simulink model "SOGI_PLL_NOFLL"  (R2020b)
settings: Solver=FixedStepDiscrete  StartTime=0.0  StopTime=1  FixedStep=1e-6  RelTol=1e-3
undefined symbols (not defined in the file): DiscIntNeverNeededParam
settings Model: Creator=gc45  LastModifiedBy=Administrator

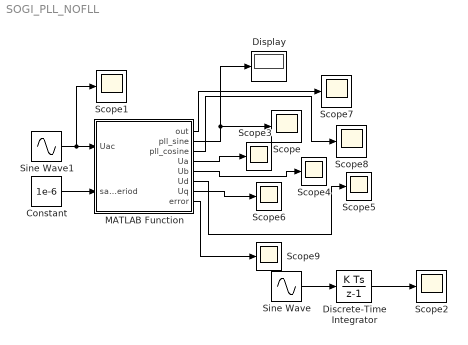
== system SOGI_PLL_NOFLL ==
  Constant : Constant  Value=1e-6
  Discrete-Time Integrator : DiscreteIntegrator  SampleTime=1e-6  ICPrevOutput=DiscIntNeverNeededParam  ICPrevScaledInput=DiscIntNeverNeededParam
  Display : Display
  MATLAB Function : MATLAB Function  TreatAsAtomicUnit=on
  Scope{,1..9} (10 alike) : Scope
  Sine Wave : Sin  Amplitude=100  Frequency=100*pi  SampleTime=1e-6
  Sine Wave1 : Sin  Amplitude=100  Frequency=100*pi  SampleTime=1e-6
  wires:
  Sine Wave1/1 -> Scope1/1, MATLAB Function/1(Uac)
  MATLAB Function/2(pll_sine) -> Display/1, Scope/1
  Constant/1 -> MATLAB Function/2(sample_period)
  Sine Wave/1 -> Discrete-Time Integrator/1
  Discrete-Time Integrator/1 -> Scope2/1
  MATLAB Function/4(Ua) -> Scope3/1
  MATLAB Function/5(Ub) -> Scope4/1
  MATLAB Function/6(Ud) -> Scope5/1
  MATLAB Function/7(Uq) -> Scope6/1
  MATLAB Function/1(out) -> Scope7/1
  MATLAB Function/3(pll_cosine) -> Scope8/1
  MATLAB Function/8(error) -> Scope9/1

== matlab function SOGI_PLL_NOFLL/MATLAB Function ==
  data: out output; Uac input; pll_sine output; sample_period input; pll_cosine output; Ua output; Ub output; Ud output; Uq output; error output
function [out,pll_sine,pll_cosine,Ua,Ub,Ud,Uq,error] = RefGen(Uac, sample_period)

%参数初始化
persistent PredictiveuAC_Intg PredictiveuAC pll_out PhaseDeviation Input_OSG;
persistent pll_Sine pll_Cosine pll_wt Vg_amp PhaseDeviation_Intg;
if isempty(pll_out)
    PredictiveuAC = 0; %Ualpha
	PredictiveuAC_Intg = 0;%Ubeta
	pll_out = 0;
	PhaseDeviation = 0;
	Input_OSG = 0;
	pll_Sine = 0;
	pll_Cosine = 0;
	pll_wt =0;
	Vg_amp = 0;
	PhaseDeviation_Intg = 0;
end
persistent Intg1 Intg2;
if isempty(Intg1)
    Intg1 = 0;
    Intg2 = 0;
end
dataType = 'double';
Kp_Predictive = 1.414;%100>>8
Ki_SOGI = 5;
Kp_SOGI = 15;
%正交信号发生器环节
   Input_OSG = (Uac-PredictiveuAC) * Kp_Predictive;
   Intg1 = (Input_OSG-PredictiveuAC_Intg) * sample_period;
   PredictiveuAC = PredictiveuAC + Intg1 * pll_out;
   Intg2 = PredictiveuAC * sample_period;
   PredictiveuAC_Intg = PredictiveuAC_Intg + Intg2 * pll_out;
%clark变换环节
   PhaseDeviation = PredictiveuAC_Intg*pll_Cosine - PredictiveuAC * pll_Sine;%q-axis
   Vg_amp = PredictiveuAC_Intg*pll_Sine + PredictiveuAC * pll_Cosine;%d-axis
%PI环节
   PhaseDeviation_Intg = PhaseDeviation_Intg + PhaseDeviation;
   pll_out = 314.159265358979 + PhaseDeviation_Intg * Ki_SOGI + PhaseDeviation * Kp_SOGI;
%限幅环节
   if(pll_out > 439)
       pll_out = 439;
   end
   if(pll_out < 251)
       pll_out = 251;
   end
   pll_wt = pll_wt + pll_out * sample_period;
   while(pll_wt > 2*pi)
       pll_wt = pll_wt - 2*pi;
   end
   while(pll_wt<0)
       pll_wt = pll_wt + 2*pi;
   end
   out = pll_out;
   pll_Sine = sin(pll_wt);
   pll_Cosine = cos(pll_wt);
   pll_sine = pll_Sine;
   pll_cosine = pll_Cosine;
   Ua = PredictiveuAC;
   Ub = PredictiveuAC_Intg;
   Ud = Vg_amp;
   Uq = PhaseDeviation;
   error = PhaseDeviation_Intg;
